simulink subsystem "IMU"  (R2021a)
settings: Solver=VariableStepAuto  StartTime=0.0  StopTime=10.0  RelTol=1e-3
undefined symbols (not defined in the file): biasAcc, biasAng, deg, euler0, rad, s
libraries: simulink x8, dspsrcs4 x6, aerolibconvert2 x2, sharedtransform x1
settings Model: Creator=jmher  LastModifiedBy=jmher

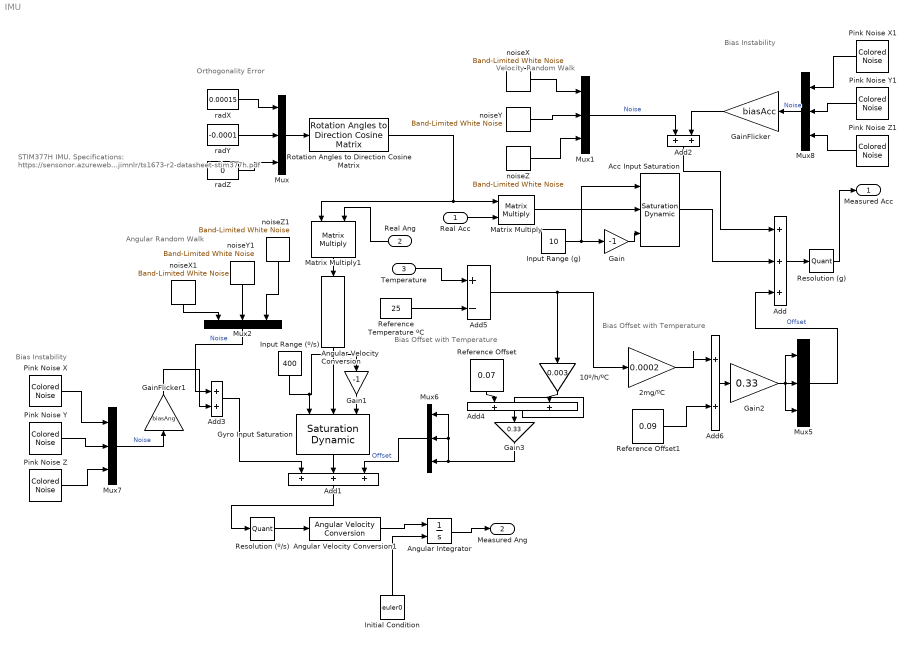
== system IMU ==
  note: Velocity Random Walk
  note: Orthogonality Error
  note: Angular Random Walk
  note: Bias Instability
  note: Bias Instability
  note: Bias Offset with Temperature
  note: Bias Offset with Temperature
  note: STIM377H IMU.
      |
      | Specifications: https://sensonor.azurewebsites.net/media/qkjimnlr/ts1673-r2-datasheet-stim377h.pdf
  Real Acc : Inport  PortDimensions=3
  Real Ang : Inport  Port=2  PortDimensions=3
  Temperature : Inport  Port=3
  10º/h/ºC : Gain  Gain=0.003
  2mg/ºC : Gain  Gain=0.0002
  Acc Input Saturation : simulink/Discontinuities/Saturation Dynamic  OutMin=[]  OutMax=[]  OutDataTypeStr=Inherit: Same as second input  OutDataType=fixdt(1, 16)  OutScaling=2^-10  DoSatur=off
  Add : Sum  Inputs=+|+|+
  Add1 : Sum  Inputs=+|+|+
  Add{2..4,6} (4 alike) : Sum  Inputs=+|+
  Add5 : Sum  Inputs=+|-
  Angular Integrator : Integrator  InitialConditionSource=external
  Angular Velocity Conversion : aerolibconvert2/Angular Velocity Conversion  IU=rad/s  OU=deg/s
  Angular Velocity Conversion1 : aerolibconvert2/Angular Velocity Conversion  IU=deg/s  OU=rad/s
  Gain : Gain  Gain=-1
  Gain1 : Gain  Gain=-1
  Gain2 : Gain  Gain=0.33
  Gain3 : Gain  Gain=0.33
  GainFlicker : Gain  Gain=biasAcc
  GainFlicker1 : Gain  Gain=biasAng
  Gyro Input Saturation : simulink/Discontinuities/Saturation Dynamic  OutMin=[]  OutMax=[]  OutDataTypeStr=Inherit: Same as second input  OutDataType=fixdt(1, 16)  OutScaling=2^-10  DoSatur=off
  Initial Condition : Constant  Value=euler0
  Input Range (g) : Constant  Value=10
  Input Range (º/s) : Constant  Value=400
  Matrix Multiply : Product  Multiplication=Matrix(*)
  Matrix Multiply1 : Product  Multiplication=Matrix(*)
  Mux{,1..2,5..8} (7 alike) : Mux  Inputs=3
  Pink Noise X : dspsrcs4/Colored Noise  Color=pink  InverseFrequencyPower=biasAcc  BoundedOutput=off  NumChannels=1  OutputDataType=double  SamplesPerFrame=1  SampleTime=1/40  RandomStream=mt19937ar with seed  Seed=12237  SimulateUsing=Interpreted execution
      settings: SourceProductBaseCode=DS
  Pink Noise X1 : dspsrcs4/Colored Noise  Color=pink  InverseFrequencyPower=biasAcc  BoundedOutput=off  NumChannels=1  OutputDataType=double  SamplesPerFrame=1  SampleTime=1/40  RandomStream=mt19937ar with seed  Seed=6237342  SimulateUsing=Interpreted execution
      settings: SourceProductBaseCode=DS
  Pink Noise Y : dspsrcs4/Colored Noise  Color=pink  InverseFrequencyPower=biasAcc  BoundedOutput=off  NumChannels=1  OutputDataType=double  SamplesPerFrame=1  SampleTime=1/40  RandomStream=mt19937ar with seed  Seed=76372  SimulateUsing=Interpreted execution
      settings: SourceProductBaseCode=DS
  Pink Noise Y1 : dspsrcs4/Colored Noise  Color=pink  InverseFrequencyPower=biasAcc  BoundedOutput=off  NumChannels=1  OutputDataType=double  SamplesPerFrame=1  SampleTime=1/40  RandomStream=mt19937ar with seed  Seed=225421  SimulateUsing=Interpreted execution
      settings: SourceProductBaseCode=DS
  Pink Noise Z : dspsrcs4/Colored Noise  Color=pink  InverseFrequencyPower=biasAcc  BoundedOutput=off  NumChannels=1  OutputDataType=double  SamplesPerFrame=1  SampleTime=1/40  RandomStream=mt19937ar with seed  Seed=3755  SimulateUsing=Interpreted execution
      settings: SourceProductBaseCode=DS
  Pink Noise Z1 : dspsrcs4/Colored Noise  Color=pink  InverseFrequencyPower=biasAcc  BoundedOutput=off  NumChannels=1  OutputDataType=double  SamplesPerFrame=1  SampleTime=1/40  RandomStream=mt19937ar with seed  Seed=345617  SimulateUsing=Interpreted execution
      settings: SourceProductBaseCode=DS
  Reference Offset : Constant  Value=0.07
  Reference Offset1 : Constant  Value=0.09
  Reference Temperature ºC : Constant  Value=25
  Resolution (g) : Quantizer  QuantizationInterval=1.9e-6  LinearizeAsGain=off
  Resolution (º/s) : Quantizer  QuantizationInterval=0.22/3600  LinearizeAsGain=off
  Rotation Angles to Direction Cosine Matrix : sharedtransform/Rotation Angles to Direction Cosine Matrix  rotationOrder=ZYX  aMode=aMode
      settings: SourceProductBaseCode=AE,PW,DR,MT,UV,VE
  noiseX : simulink/Sources/Band-Limited White Noise  Cov=noiseAcc  Ts=1/40  seed=[32323556]
  noiseX1 : simulink/Sources/Band-Limited White Noise  Cov=noiseAng  Ts=1/40  seed=[3256]
  noiseY : simulink/Sources/Band-Limited White Noise  Cov=noiseAcc  Ts=1/40  seed=[238641]
  noiseY1 : simulink/Sources/Band-Limited White Noise  Cov=noiseAng  Ts=1/40  seed=[567380]
  noiseZ : simulink/Sources/Band-Limited White Noise  Cov=noiseAcc  Ts=1/40  seed=[23341231]
  noiseZ1 : simulink/Sources/Band-Limited White Noise  Cov=noiseAng  Ts=1/40  seed=[234234111]
  radX : Constant  Value=0.00015
  radY : Constant  Value=-0.0001
  radZ : Constant  Value=0
  Measured Acc : Outport  SampleTime=1/40
  Measured Ang : Outport  Port=2  SampleTime=1/40
  wires:
  noiseY/1 -> Mux1/2
  Acc Input Saturation/1 -> Add/2
  Add/1 -> Resolution (g)/1
  noiseZ/1 -> Mux1/3
  noiseX/1 -> Mux1/1
  Gain/1 -> Acc Input Saturation/3
  Gain1/1 -> Gyro Input Saturation/3
  Input Range (g)/1 -> Acc Input Saturation/1, Gain/1
  radY/1 -> Mux/2
  Mux/1 -> Rotation Angles to Direction Cosine Matrix/1
  radX/1 -> Mux/1
  radZ/1 -> Mux/3
  Rotation Angles to Direction Cosine Matrix/1 -> Matrix Multiply/1, Matrix Multiply1/1
  Real Acc/1 -> Matrix Multiply/2
  Matrix Multiply/1 -> Acc Input Saturation/2
  Gyro Input Saturation/1 -> Add1/2
  Add1/1 -> Resolution (º/s)/1
  noiseY1/1 -> Mux2/2
  noiseZ1/1 -> Mux2/3
  noiseX1/1 -> Mux2/1
  Mux1/1 -> Add2/1  "Noise"
  Input Range (º/s)/1 -> Gyro Input Saturation/1, Gain1/1
  Mux2/1 -> Add3/1  "Noise"
  Add3/1 -> Add1/1
  GainFlicker/1 -> Add2/2
  GainFlicker1/1 -> Add3/2
  Reference Offset/1 -> Add4/1
  Add2/1 -> Add/1
  Reference Offset1/1 -> Add6/2
  Add5/1 -> 10º/h/ºC/1, 2mg/ºC/1
  Temperature/1 -> Add5/1
  Reference Temperature ºC/1 -> Add5/2
  2mg/ºC/1 -> Add6/1
  Angular Velocity Conversion/1 -> Gyro Input Saturation/2
  Resolution (º/s)/1 -> Angular Velocity Conversion1/1
  Add6/1 -> Gain2/1
  Mux5/1 -> Add/3  "Offset"
  Gain3/1 -> Mux6/1, Mux6/2, Mux6/3
  Add4/1 -> Gain3/1
  Mux6/1 -> Add1/3  "Offset"
  Gain2/1 -> Mux5/1, Mux5/3, Mux5/2
  Pink Noise X/1 -> Mux7/1
  Pink Noise Y/1 -> Mux7/2
  Pink Noise Z/1 -> Mux7/3
  Mux7/1 -> GainFlicker1/1  "Noise"
  Pink Noise Y1/1 -> Mux8/2
  Pink Noise Z1/1 -> Mux8/3
  Pink Noise X1/1 -> Mux8/1
  Mux8/1 -> GainFlicker/1  "Noise"
  Angular Integrator/1 -> Measured Ang/1
  Angular Velocity Conversion1/1 -> Angular Integrator/1
  Real Ang/1 -> Matrix Multiply1/2
  Matrix Multiply1/1 -> Angular Velocity Conversion/1
  Resolution (g)/1 -> Measured Acc/1
  10º/h/ºC/1 -> Add4/2
  Initial Condition/1 -> Angular Integrator/2
